simulink model "Frdm_ver1"  (R2016b)
settings: Solver=FixedStepDiscrete  StartTime=0.0  StopTime=10.0  RelTol=1e-3  EnableMultiTasking=on
undefined symbols (not defined in the file): D0, D1, PTA1, PTA2
libraries: simulink x6, frdmtfcshieldlib x5, frdmkl25zlib x2, slrtlib x2
settings Model: ExtModeTrigDuration=5  Creator=jays  LastModifiedBy=jays
settings OptimizationCC: MaxStackSize=64
settings DebuggingCC: ParameterTunabilityLossMsg=error
settings HardwareCC: ProdBitPerPointer=32  ProdBitPerSizeT=32  ProdBitPerPtrDiffT=32  ProdLargestAtomicInteger=Long  ProdLargestAtomicFloat=Double  ProdWordSize=32  ProdHWDeviceType=ARM Compatible->ARM Cortex
settings RTWCC: SystemTargetFile=ert.tlc  HardwareBoard=NXP FRDM-KL25Z  TLCOptions=-aInlineSetEventsForThisBaseRateFcn=TLC_FALSE -aSuppressMultiTaskScheduler=TLC_FALSE -aRateBasedStepFcn=1  TemplateMakefile=ert_default_tmf  Description=Embedded Coder  GenerateReport=on  Toolchain=GNU Tools for ARM Embedded Processors  IncludeHyperlinkInReport=on  LaunchReport=on  GenerateTraceInfo=on  GenerateTraceReport=on  GenerateTraceReportSl=on  GenerateTraceReportSf=on  GenerateTraceReportEml=on
settings CodeAppCC: ForceParamTrailComments=on  IgnoreCustomStorageClasses=off  OperatorAnnotations=on  SimulinkDataObjDesc=on  SFDataObjDesc=on  MATLABFcnDesc=on  InsertBlockDesc=on  MATLABSourceComments=on

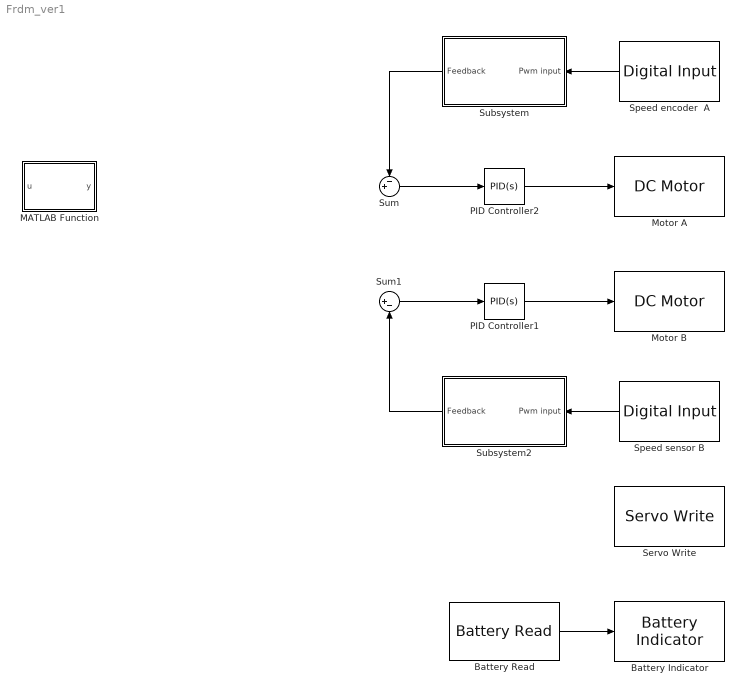
== system Frdm_ver1 ==
  Battery Indicator : frdmtfcshieldlib/Battery Indicator
  Battery Read : frdmtfcshieldlib/Battery Read  SampleTime=0.1
  MATLAB Function : MATLAB Function  TreatAsAtomicUnit=on
  Motor A : frdmtfcshieldlib/DC Motor  WhichMotor=A
  Motor B : frdmtfcshieldlib/DC Motor  WhichMotor=B
  PID Controller1 : simulink/Continuous/PID Controller  Controller=PID  TimeDomain=Continuous-time  SampleTime=-1  IntegratorMethod=Forward Euler  FilterMethod=Forward Euler  Form=Parallel  UseFilter=on  ControllerParametersSource=internal  P=1  I=1  D=0  N=100  InitialConditionSource=internal  InitialConditionForIntegrator=0  InitialConditionForFilter=0  ExternalReset=none  LimitOutput=off  UpperSaturationLimit=inf  LowerSaturationLimit=-inf  LinearizeAsGain=on  AntiWindupMode=none  Kb=1  TrackingMode=off  Kt=1  PParamMin=[]  PParamMax=[]  IParamMin=[]  IParamMax=[]  DParamMin=[]  DParamMax=[]  NParamMin=[]  NParamMax=[]  KbParamMin=[]  KbParamMax=[]  KtParamMin=[]  KtParamMax=[]  POutMin=[]  POutMax=[]  IOutMin=[]  IOutMax=[]  DOutMin=[]  DOutMax=[]  NOutMin=[]  NOutMax=[]  KbOutMin=[]  KbOutMax=[]  KtOutMin=[]  KtOutMax=[]  IntegratorOutMin=[]  IntegratorOutMax=[]  FilterOutMin=[]  FilterOutMax=[]  SumOutMin=[]  SumOutMax=[]  SumI1OutMin=[]  SumI1OutMax=[]  SumI2OutMin=[]  SumI2OutMax=[]  SumI3OutMin=[]  SumI3OutMax=[]  SumDOutMin=[]  SumDOutMax=[]  SaturationOutMin=[]  SaturationOutMax=[]  IntegratorContinuousStateAttributes=''  IntegratorStateMustResolveToSignalObject=off  IntegratorRTWStateStorageClass=Auto  FilterContinuousStateAttributes=''  FilterStateMustResolveToSignalObject=off  FilterRTWStateStorageClass=Auto  DifferentiatorICPrevScaledInput=0  DifferentiatorOutMin=[]  DifferentiatorOutMax=[]
  PID Controller2 : simulink/Continuous/PID Controller  Controller=PID  TimeDomain=Continuous-time  SampleTime=-1  IntegratorMethod=Forward Euler  FilterMethod=Forward Euler  Form=Parallel  UseFilter=on  ControllerParametersSource=internal  P=1  I=1  D=0  N=100  InitialConditionSource=internal  InitialConditionForIntegrator=0  InitialConditionForFilter=0  ExternalReset=none  LimitOutput=off  UpperSaturationLimit=inf  LowerSaturationLimit=-inf  LinearizeAsGain=on  AntiWindupMode=none  Kb=1  TrackingMode=off  Kt=1  PParamMin=[]  PParamMax=[]  IParamMin=[]  IParamMax=[]  DParamMin=[]  DParamMax=[]  NParamMin=[]  NParamMax=[]  KbParamMin=[]  KbParamMax=[]  KtParamMin=[]  KtParamMax=[]  POutMin=[]  POutMax=[]  IOutMin=[]  IOutMax=[]  DOutMin=[]  DOutMax=[]  NOutMin=[]  NOutMax=[]  KbOutMin=[]  KbOutMax=[]  KtOutMin=[]  KtOutMax=[]  IntegratorOutMin=[]  IntegratorOutMax=[]  FilterOutMin=[]  FilterOutMax=[]  SumOutMin=[]  SumOutMax=[]  SumI1OutMin=[]  SumI1OutMax=[]  SumI2OutMin=[]  SumI2OutMax=[]  SumI3OutMin=[]  SumI3OutMax=[]  SumDOutMin=[]  SumDOutMax=[]  SaturationOutMin=[]  SaturationOutMax=[]  IntegratorContinuousStateAttributes=''  IntegratorStateMustResolveToSignalObject=off  IntegratorRTWStateStorageClass=Auto  FilterContinuousStateAttributes=''  FilterStateMustResolveToSignalObject=off  FilterRTWStateStorageClass=Auto  DifferentiatorICPrevScaledInput=0  DifferentiatorOutMin=[]  DifferentiatorOutMax=[]
  Servo Write : frdmtfcshieldlib/Servo Write  WhichServo=0  minAngle=-20.0  maxAngle=20.0
  Speed encoder  A : frdmkl25zlib/Digital Input  Priority=2  WhichPin=PTA1 (D0)  SampleTime=0.0001
  Speed sensor B : frdmkl25zlib/Digital Input  Priority=2  WhichPin=PTA2 (D1)  SampleTime=0.1
  Subsystem : Subsystem
  Subsystem2 : Subsystem
  Sum : Sum  Inputs=-+|
  Sum1 : Sum  Inputs=|+-
  wires:
  PID Controller2/1 -> Motor A/1
  PID Controller1/1 -> Motor B/1
  Sum1/1 -> PID Controller1/1
  Sum/1 -> PID Controller2/1
  ? -> Sum1/1, Sum/2
  ? -> Servo Write/1
  Battery Read/1 -> Battery Indicator/1
  Speed encoder  A/1 -> Subsystem/1(Pwm input)
  Subsystem/1(Feedback) -> Sum/1
  Speed sensor B/1 -> Subsystem2/1(Pwm input)
  Subsystem2/1(Feedback) -> Sum1/2

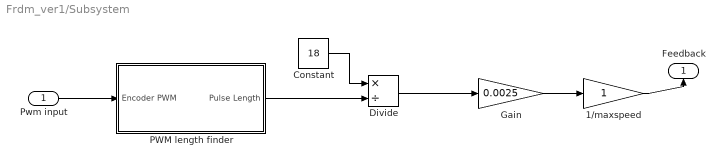
== system Frdm_ver1/Subsystem ==
  Pwm input : Inport
  1/maxspeed : Gain
  Constant : Constant  Value=18
  Divide : Product  Inputs=*/
  Gain : Gain  Gain=0.0025
  PWM length finder : Subsystem
  Feedback : Outport
  wires:
  PWM length finder/1(Pulse Length) -> Divide/2
  Pwm input/1 -> PWM length finder/1(Encoder PWM)
  Gain/1 -> 1/maxspeed/1
  Constant/1 -> Divide/1
  Divide/1 -> Gain/1
  1/maxspeed/1 -> Feedback/1

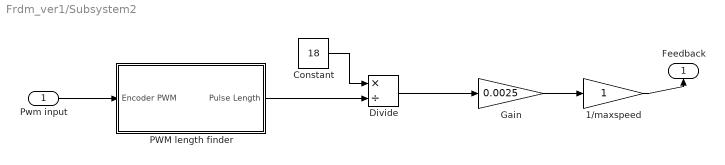
== system Frdm_ver1/Subsystem2 ==
  Pwm input : Inport
  1/maxspeed : Gain
  Constant : Constant  Value=18
  Divide : Product  Inputs=*/
  Gain : Gain  Gain=0.0025
  PWM length finder : Subsystem
  Feedback : Outport
  wires:
  PWM length finder/1(Pulse Length) -> Divide/2
  Pwm input/1 -> PWM length finder/1(Encoder PWM)
  Gain/1 -> 1/maxspeed/1
  Constant/1 -> Divide/1
  Divide/1 -> Gain/1
  1/maxspeed/1 -> Feedback/1

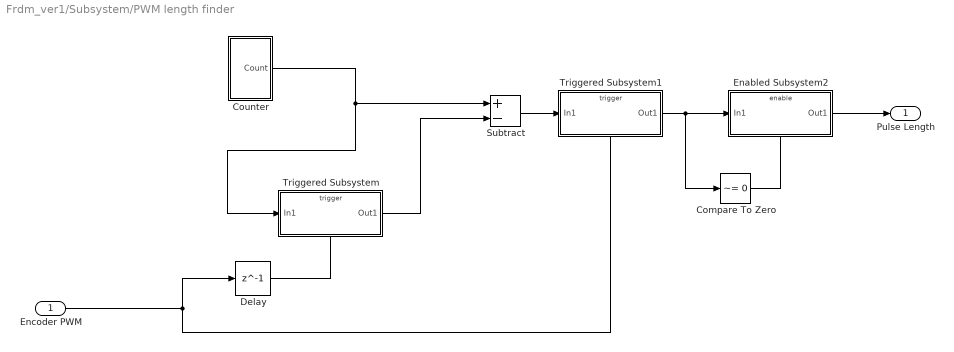
== system Frdm_ver1/Subsystem/PWM length finder ==
  Encoder PWM : Inport
  Compare To Zero : simulink/Logic and Bit Operations/Compare To Zero  relop=~=  OutDataTypeStr=boolean
  "Counter " : Subsystem
  Delay : Delay  DelayLength=1  InitialCondition=0  SampleTime=0.0001
  Enabled Subsystem2 : Subsystem  TreatAsAtomicUnit=on
  Subtract : Sum  Inputs=+-
  Triggered Subsystem : Subsystem  TreatAsAtomicUnit=on
  Triggered Subsystem1 : Subsystem  TreatAsAtomicUnit=on
  Pulse Length : Outport
  wires:
  Delay/1 -> Triggered Subsystem/Trigger
  Encoder PWM/1 -> Delay/1, Triggered Subsystem1/Trigger
  Compare To Zero/1 -> Enabled Subsystem2/Enable
  Enabled Subsystem2/1(Out1) -> Pulse Length/1
  Triggered Subsystem1/1(Out1) -> Compare To Zero/1, Enabled Subsystem2/1(In1)
  Triggered Subsystem/1(Out1) -> Subtract/2
  "Counter "/1(Count) -> Subtract/1, Triggered Subsystem/1(In1)
  Subtract/1 -> Triggered Subsystem1/1(In1)

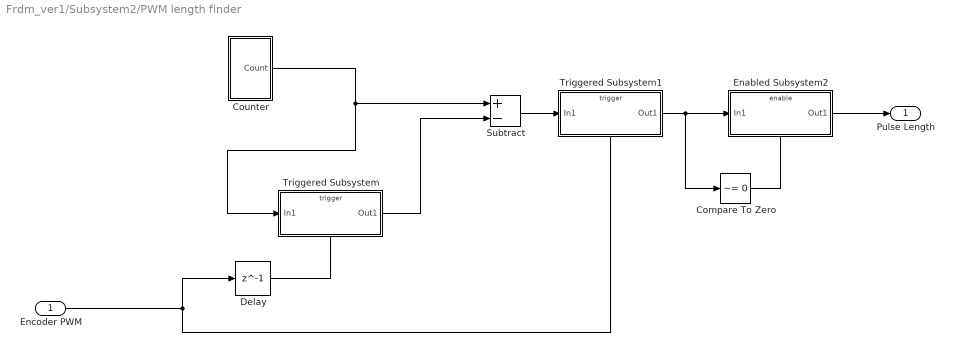
== system Frdm_ver1/Subsystem2/PWM length finder ==
  Encoder PWM : Inport
  Compare To Zero : simulink/Logic and Bit Operations/Compare To Zero  relop=~=  OutDataTypeStr=boolean
  "Counter " : Subsystem
  Delay : Delay  DelayLength=1  InitialCondition=0  SampleTime=0.0001
  Enabled Subsystem2 : Subsystem  TreatAsAtomicUnit=on
  Subtract : Sum  Inputs=+-
  Triggered Subsystem : Subsystem  TreatAsAtomicUnit=on
  Triggered Subsystem1 : Subsystem  TreatAsAtomicUnit=on
  Pulse Length : Outport
  wires:
  Delay/1 -> Triggered Subsystem/Trigger
  Encoder PWM/1 -> Delay/1, Triggered Subsystem1/Trigger
  Compare To Zero/1 -> Enabled Subsystem2/Enable
  Enabled Subsystem2/1(Out1) -> Pulse Length/1
  Triggered Subsystem1/1(Out1) -> Compare To Zero/1, Enabled Subsystem2/1(In1)
  Triggered Subsystem/1(Out1) -> Subtract/2
  "Counter "/1(Count) -> Subtract/1, Triggered Subsystem/1(In1)
  Subtract/1 -> Triggered Subsystem1/1(In1)

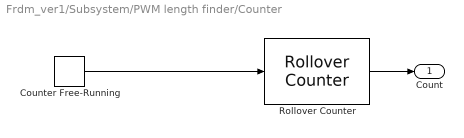
== system Frdm_ver1/Subsystem/PWM length finder/Counter  ==
  Counter Free-Running : simulink/Sources/Counter Free-Running  NumBits=16  tsamp=0.0001
  "Rollover Counter " : slrtlib/Incremental Encoder/Utilities/Rollover/Rollover Counter   InitialValue=0  RolloverThreshold=2^15
  Count : Outport
  wires:
  Counter Free-Running/1 -> "Rollover Counter "/1
  "Rollover Counter "/1 -> Count/1

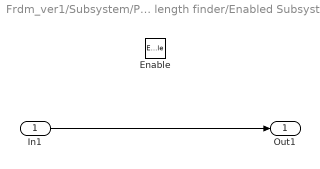
== system Frdm_ver1/Subsystem/PWM length finder/Enabled Subsystem2 ==
  In1 : Inport
  Enable : EnablePort
  Out1 : Outport
  wires:
  In1/1 -> Out1/1

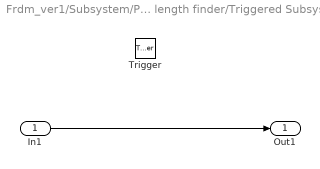
== system Frdm_ver1/Subsystem/PWM length finder/Triggered Subsystem ==
  In1 : Inport
  Trigger : TriggerPort  VariantControl=Variant
  Out1 : Outport
  wires:
  In1/1 -> Out1/1

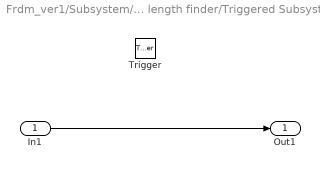
== system Frdm_ver1/Subsystem/PWM length finder/Triggered Subsystem1 ==
  In1 : Inport
  Trigger : TriggerPort  VariantControl=Variant
  Out1 : Outport
  wires:
  In1/1 -> Out1/1

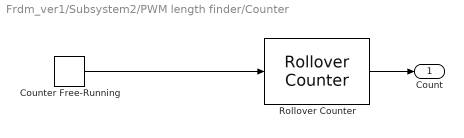
== system Frdm_ver1/Subsystem2/PWM length finder/Counter  ==
  Counter Free-Running : simulink/Sources/Counter Free-Running  NumBits=16  tsamp=0.0001
  "Rollover Counter " : slrtlib/Incremental Encoder/Utilities/Rollover/Rollover Counter   InitialValue=0  RolloverThreshold=2^15
  Count : Outport
  wires:
  Counter Free-Running/1 -> "Rollover Counter "/1
  "Rollover Counter "/1 -> Count/1

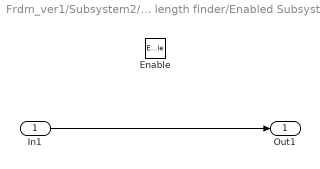
== system Frdm_ver1/Subsystem2/PWM length finder/Enabled Subsystem2 ==
  In1 : Inport
  Enable : EnablePort
  Out1 : Outport
  wires:
  In1/1 -> Out1/1

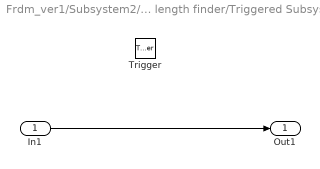
== system Frdm_ver1/Subsystem2/PWM length finder/Triggered Subsystem ==
  In1 : Inport
  Trigger : TriggerPort  VariantControl=Variant
  Out1 : Outport
  wires:
  In1/1 -> Out1/1

== system Frdm_ver1/Subsystem2/PWM length finder/Triggered Subsystem1 ==
  In1 : Inport
  Trigger : TriggerPort  VariantControl=Variant
  Out1 : Outport
  wires:
  In1/1 -> Out1/1

== matlab function Frdm_ver1/MATLAB Function ==
  data: u input; y output
function y = fcn(u)
#include <stdlib.h>

#include "serial_port.h"

int main(int argc, char *argv[])
{
    if(argc < 3)
    {
        return 1;
    }

    const char *dev = argv[1];
    const char *baud_rate_string = argv[2];
    const int baud_rate = atoi(baud_rate_string);

    int file_description;

    file_description = open_serial_port(dev);

    if(file_description == -1)
    {
        return 1;
    }

    if(set_port_attribute(file_description, baud_rate))
    {
        return 1;
    }

    close(file_description);

    return 0;
}
